simulink model "ddc_bpm_476_066_hw_cosim"  (Simulink 7.8)
settings: Solver=ode45  StartTime=0.0  StopTime=200e-4  RelTol=1e-3
undefined symbols (not defined in the file): A, dt_sim, frev_476, Fs_adc, N
libraries: simulink x3, xbsIndex_r4 x1, JTAGRuntimeCosim_r4 x1
settings Model: Creator=lucas.russo  LastModifiedBy=lucas.russo

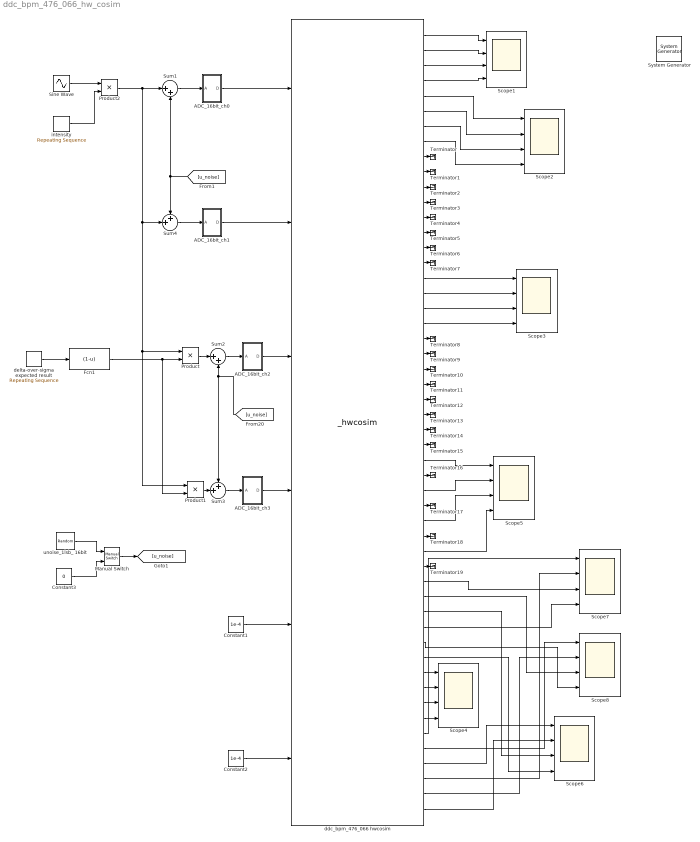
== system ddc_bpm_476_066_hw_cosim ==
  " System Generator" : xbsIndex_r4/ System Generator  Tag=genX  xilinxfamily=virtex6  part=xc6vlx240t  speed=-1  package=ff1156  synthesis_tool=XST  clock_wrapper=Clock Enables  directory=./netlistJTAG_COsim_ddc_bpm_476_066  proj_type=Project Navigator  Synth_file=XST Defaults  Impl_file=ISE Defaults  testbench=on  simulink_period=dt_sim  sysclk_period=10  dcm_input_clock_period=10  incr_netlist=off  trim_vbits=Everywhere in SubSystem  dbl_ovrd=According to Block Masks  core_generation=According to Block Masks  run_coregen=off  deprecated_control=off  eval_field=0  block_type=sysgen
  ADC_16bit_ch0 : Subsystem
  ADC_16bit_ch1 : Subsystem
  ADC_16bit_ch2 : Subsystem
  ADC_16bit_ch3 : Subsystem
  Constant1 : Constant  Value=1e-4  OutDataTypeStr=fixdt(1,26,22)
  Constant2 : Constant  Value=1e-4  OutDataTypeStr=fixdt(1,26,22)
  Constant3 : Constant  Value=0  SampleTime=0
  Fcn1 : Fcn  Expr=(1-u)
  Manual Switch : simulink/Signal Routing/Manual Switch  sw=1  action=0  varsize=off
  Product : Product  RndMeth=Zero
  Product1 : Product  RndMeth=Zero
  Product2 : Product  RndMeth=Zero
  Scope{1..8} (8 alike) : Scope  NumInputPorts=4
      Scope1 settings: TimeRange=4.726537192257835e-007  YMin=4.34876e-005~0.463882~0.00990226~4.5e-005  YMax=4.80652e-005~0.512712~0.0111025~9.5e-005  MaxDataPoints=1000000
      Scope2 settings: TimeRange=4.726537192257835e-007  YMin=4.34876e-005~0.463882~0.00990226~4.5e-005  YMax=4.80652e-005~0.512712~0.0111025~9.5e-005  MaxDataPoints=1000000
      Scope3 settings: TimeRange=4.726537192257835e-007  YMin=4.34876e-005~0.463882~0.00990226~4.5e-005  YMax=4.80652e-005~0.512712~0.0111025~9.5e-005  SaveName=ScopeData2  MaxDataPoints=1000000
      Scope4 settings: TimeRange=4.726537192257835e-007  YMin=4.34876e-005~0.463882~0.00990226~4.5e-005  YMax=4.80652e-005~0.512712~0.0111025~9.5e-005  SaveName=ScopeData3  MaxDataPoints=1000000
      Scope5 settings: TimeRange=4.726537192257835e-007  YMin=4.34876e-005~0.463882~0.00990226~4.5e-005  YMax=4.80652e-005~0.512712~0.0111025~9.5e-005  SaveName=ScopeData4  MaxDataPoints=1000000
      Scope6 settings: TimeRange=4.726537192257835e-007  YMin=4.34876e-005~0.463882~0.00990226~4.5e-005  YMax=4.80652e-005~0.512712~0.0111025~9.5e-005  SaveName=ScopeData5  MaxDataPoints=1000000
      Scope7 settings: TimeRange=4.726537192257835e-007  YMin=4.34876e-005~1.14441e-005~0.00990226~4.5e-005  YMax=4.80652e-005~1.14441e-005~0.0111025~9.5e-005  SaveName=ScopeData6  MaxDataPoints=1000000
      Scope8 settings: TimeRange=4.726537192257835e-007  YMin=4.34876e-005~-3.75509e-007~0.00990226~4.5e-005  YMax=4.80652e-005~-3.39747e-007~0.0111025~9.5e-005  SaveName=ScopeData7  MaxDataPoints=1000000
  Sine Wave : Sin  Frequency=2*pi*frev_476  SampleTime=0
  Sum1 : Sum  Inputs=|++
  Sum2 : Sum  Inputs=|++
  Sum3 : Sum  Inputs=++|
  Sum4 : Sum  Inputs=++|
  Terminator{,1..19} (20 alike) : Terminator
  ddc_bpm_476_066 hwcosim : JTAGRuntimeCosim_r4/_hwcosim  clkSrc=Single Stepped  hasCombinationalPath=on  bitfileName=D:\Sysgen_projects\ddc_bpm_476_066\models\netlistJTAG_COsim_ddc_bpm_476_066_v2_3\ddc_bpm_476_066_cw.bit  skipConfig=off  cable=Auto Detect  speed=N/A  cablePort=N/A  cableLocation=Local  shareCable=off  enable_codebug=on  design_xtable=|  engineDll=JTAGCosimEngine.dll  cableWaitTime=10  bscanPos=-1  IRLengths=[]  useWaitBox=1  hasBufgmux=on  Scheme=Cosim  useCmdProc=1  hasProc=0  block_type=jtagcosim
      | {
      |   'clkWrapper' => 'ddc_bpm_476_066_cw',
      |   'clocksGcd' => 1,
      |   'device' => 'xc6vlx240t-1ff1156',
      |   'ports' => {
      |     'adc_ch0_dbg_data_o' => {
      |       'bd_port_index' => 0,
      |       'direction' => 'out',
      |       'icon_text' => 'adc_ch0_dbg_data_o',
      |       'period' => 1,
      |       'proxy_name' => 'ddc_bpm_476_066/BPF/adc_ch0_dbg_data_o',
      |       'sim_pause_trigger' => false,
      |       'type' => 'Fix_16_15',
      |       'width' => 16,
      |     },
      |     'adc_ch0_i' => {
      |       'bd_port_index' => 0,
      |       'direction' => 'in',
      |       'icon_text' => 'adc_ch0_i',
      |       'period' => 1,
      |       'proxy_name' => 'ddc_bpm_476_066/adc_ch0_i',
      |       'sim_pause_trigger' => false,
      |       'type' => 'Fix_16_15',
      |       'width' => 16,
      |     },
      |     'adc_ch1_dbg_data_o' => {
      |       'bd_port_index' => 1,
      |       'direction' => 'out',
      |       'icon_text' => 'adc_ch1_dbg_data_o',
      |       'period' => 1,
      |       'proxy_name' => 'ddc_bpm_476_066/BPF/adc_ch1_dbg_data_o',
      |       'sim_pause_trigger' => false,
      |       'type' => 'Fix_16_15',
      |       'width' => 16,
      |     },
      |     'adc_ch1_i' => {
      |       'bd_port_index' => 1,
      |       'direction' => 'in',
      |       'icon_text' => 'adc_ch1_i',
      |       'period' => 1,
      |       'proxy_name' => 'ddc_bpm_476_066/adc_ch1_i',
      |       'sim_pause_trigger' => false,
      |       'type' => 'Fix_16_15',
      |       'width' => 16,
      |     },
      |     'adc_ch2_dbg_data_o' => {
      |       'bd_port_index' => 2,
      |       'direction' => 'out',
      |       'icon_text' => 'adc_ch2_dbg_data_o',
      |       'period' => 1,
      |       'proxy_name' => 'ddc_bpm_476_066/BPF/adc_ch2_dbg_data_o',
      |       'sim_pause_trigger' => false,
      |       'type' => 'Fix_16_15',
      |       'width' => 16,
      |     },
      |     'adc_ch2_i' => {
      |       'bd_port_index' => 2,
      |       'direction' => 'in',
      |       'icon_text' => 'adc_ch2_i',
      |       'period' => 1,
      |       'proxy_name' => 'ddc_bpm_476_066/adc_ch2_i',
      |       'sim_pause_trigger' => false,
      |       'type' => 'Fix_16_15',
      |       'width' => 16,
      |     },
      |     'adc_ch3_dbg_data_o' => {
      |       'bd_port_index' => 3,
      |       'direction' => 'out',
      |       'icon_text' => 'adc_ch3_dbg_data_o',
      |       'period' => 1,
      |       'proxy_name' => 'ddc_bpm_476_066/BPF/adc_ch3_dbg_data_o',
      |       'sim_pause_trigger' => false,
      |       'type' => 'Fix_16_15',
      |       'width' => 16,
      |     },
      |     'adc_ch3_i' => {
      |       'bd_port_index' => 3,
      |       'direction' => 'in',
      |       'icon_text' => 'adc_ch3_i',
      |       'period' => 1,
      |       'proxy_name' => 'ddc_bpm_476_066/adc_ch3_i',
      |       'sim_pause_trigger' => false,
      |       'type' => 'Fix_16_15',
      |       'width' => 16,
      |     },
      |     'bpf_ch0_o' => {
      |       'bd_port_index' => 4,
      |       'direction' => 'out',
      |       'icon_text' => 'bpf_ch0_o',
      |       'period' => 1,
      |       'proxy_name' => 'ddc_bpm_476_066/BPF/bpf_ch0_o',
      |       'sim_pause_trigger' => false,
      |       'type' => 'Fix_24_22',
      |       'width' => 24,
      |     },
      |     'bpf_ch1_o' => {
      |       'bd_port_index' => 5,
      |       'direction' => 'out',
      |       'icon_text' => 'bpf_ch1_o',
      |       'period' => 1,
      |       'proxy_name' => 'ddc_bpm_476_066/BPF/bpf_ch1_o',
      |       'sim_pause_trigger' => false,
      |       'type' => 'Fix_24_22',
      |       'width' => 24,
      |     },
      |     'bpf_ch2_o' => {
      |       'bd_port_index' => 6,
      |       'direction' => 'out',
      |       'icon_text' => 'bpf_ch2_o',
      |       'period' => 1,
      |       'proxy_name' => 'ddc_bpm_476_066/BPF/bpf_ch2_o',
      |       'sim_pause_trigger' => false,
      |       'type' => 'Fix_24_22',
      |       'width' => 24,
      |     },
      |     'bpf_ch3_o' => {
      |       'bd_port_index' => 7,
      |       'direction' => 'out',
      |       'icon_text' => 'bpf_ch3_o',
      |       'period' => 1,
      |       'proxy_name' => 'ddc_bpm_476_066/BPF/bpf_ch3_o',
      |       'sim_pause_trigger' => false,
      |       'type' => 'Fix_24_22',
      |       'width' => 24,
      |     },
      |     'cic_fofb_ch0_i_o' => {
      |       'bd_port_index' => 8,
      |       'direction' => 'out',
      |       'icon_text' => 'cic_fofb_ch0_i_o',
      |       'period' => 1113,
      |       'proxy_name' => 'ddc_bpm_476_066/Channel0_fofb/cic_fofb_ch0_i_o',
      |       'sim_pause_trigger' => false,
      |       'type' => 'Fix_25_23',
      |       'width' => 25,
      |     },
      |     'cic_fofb_ch0_q_o' => {
      |       'bd_port_index' => 9,
      |       'direction' => 'out',
      |       'icon_text' => 'cic_fofb_ch0_q_o',
      |       'period' => 1113,
      |       'proxy_name' => 'ddc_bpm_476_066/Channel0_fofb/cic_fofb_ch0_q_o',
      |       'sim_pause_trigger' => false,
      |       'type' => 'Fix_25_23',
      |       'width' => 25,
      |     },
      |     'cic_fofb_ch1_i_o' => {
      |       'bd_port_index' => 10,
      |       'direction' => 'out',
      |       'icon_text' => 'cic_fofb_ch1_i_o',
      |       'period' => 1113,
      |       'proxy_name' => 'ddc_bpm_476_066/Channel1_fofb/cic_fofb_ch1_i_o',
      |       'sim_pause_trigger' => false,
      |       'type' => 'Fix_25_23',
      |       'width' => 25,
      |     },
      |     'cic_fofb_ch1_q_o' => {
      |       'bd_port_index' => 11,
      |       'direction' => 'out',
      |       'icon_text' => 'cic_fofb_ch1_q_o',
      |       'period' => 1113,
      |       'proxy_name' => 'ddc_bpm_476_066/Channel1_fofb/cic_fofb_ch1_q_o',
      |       'sim_pause_trigger' => false,
      |       'type' => 'Fix_25_23',
      |       'width' => 25,
      |     },
      |     'cic_fofb_ch2_i_o' => {
      |       'bd_port_index' => 12,
      |       'direction' => 'out',
      |       'icon_text' => 'cic_fofb_ch2_i_o',
      |       'period' => 1113,
      |       'proxy_name' => 'ddc_bpm_476_066/Channel2_fofb/cic_fofb_ch2_i_o',
      |       'sim_pause_trigger' => false,
      |       'type' => 'Fix_25_23',
      |       'width' => 25,
      |     },
      |     'cic_fofb_ch2_q_o' => {
      |       'bd_port_index' => 13,
      |       'direction' => 'out',
      |       'icon_text' => 'cic_fofb_ch2_q_o',
      |       'period' => 1113,
      |       'proxy_name' => 'ddc_bpm_476_066/Channel2_fofb/cic_fofb_ch2_q_o',
      |       'sim_pause_trigger' => false,
      |       'type' => 'Fix_25_23',
      |       'width' => 25,
      |     },
      |     'cic_fofb_ch3_i_o' => {
      |       'bd_port_index' => 14,
      |       'direction' => 'out',
      |       'icon_text' => 'cic_fofb_ch3_i_o',
      |       'period' => 1113,
      |       'proxy_name' => 'ddc_bpm_476_066/Channel3_fofb/cic_fofb_ch3_i_o',
      |       'sim_pause_trigger' => false,
      |       'type' => 'Fix_25_23',
      |       'width' => 25,
      |     },
      |     'cic_fofb_ch3_q_o' => {
      |       'bd_port_index' => 15,
      |       'direction' => 'out',
      |       'icon_text' => 'cic_fofb_ch3_q_o',
      |       'period' => 1113,
      |       'proxy_name' => 'ddc_bpm_476_066/Channel3_fofb/cic_fofb_ch3_q_o',
      |       'sim_pause_trigger' => false,
      |       'type' => 'Fix_25_23',
      |       'width' => 25,
      |     },
      |     'del_sig_div_fofb_thres_i' => {
      |       'bd_port_index' => 4,
      |       'direction' => 'in',
      |       'icon_text' => 'del_sig_div_fofb_thres_i',
      |       'period' => 1,
      |       'proxy_name' => 'ddc_bpm_476_066/del_sig_div_fofb_thres_i',
      |       'sim_pause_trigger' => false,
      |       'type' => 'Fix_27_23',
      |       'width' => 27,
      |     },
      |     'del_sig_div_tbt_thres_i' => {
      |       'bd_port_index' => 5,
      |       'direction' => 'in',
      |       'icon_text' => 'del_sig_div_tbt_thres_i',
      |       'period' => 1,
      |       'proxy_name' => 'ddc_bpm_476_066/del_sig_div_tbt_thres_i',
      |       'sim_pause_trigger' => false,
      |       'type' => 'Fix_27_23',
      |       'width' => 27,
      |     },
      |     'fofb_amp_ch0_o' => {
      |       'bd_port_index' => 16,
      |       'direction' => 'out',
      |       'icon_text' => 'fofb_amp_ch0_o',
      |       'period' => 1113,
      |       'proxy_name' => 'ddc_bpm_476_066/Channel0_fofb/fofb_amp_ch0_o',
      |       'sim_pause_trigger' => false,
      |       'type' => 'Fix_25_23',
      |       'width' => 25,
      |     },
      |     'fofb_amp_ch1_o' => {
      |       'bd_port_index' => 17,
      |       'direction' => 'out',
      |       'icon_text' => 'fofb_amp_ch1_o',
      |       'period' => 1113,
      |       'proxy_name' => 'ddc_bpm_476_066/Channel1_fofb/fofb_amp_ch1_o',
      |       'sim_pause_trigger' => false,
      |       'type' => 'Fix_25_23',
      |       'width' => 25,
      |     },
      |     'fofb_amp_ch2_o' => {
      |       'bd_port_index' => 18,
      |       'direction' => 'out',
      |       'icon_text' => 'fofb_amp_ch2_o',
      |       'period' => 1113,
      |       'proxy_name' => 'ddc_bpm_476_066/Channel2_fofb/fofb_amp_ch2_o',
      |       'sim_pause_trigger' => false,
      |       'type' => 'Fix_25_23',
      |       'width' => 25,
      |     },
      |     'fofb_amp_ch3_o' => {
      |       'bd_port_index' => 19,
      |       'direction' => 'out',
      |       'icon_text' => 'fofb_amp_ch3_o',
      |       'period' => 1113,
      |       'proxy_name' => 'ddc_bpm_476_066/Channel3_fofb/fofb_amp_ch3_o',
      |       'sim_pause_trigger' => false,
      |       'type' => 'Fix_25_23',
      |       'width' => 25,
      |     },
      |     'mix_ch0_i_o' => {
      |       'bd_port_index' => 20,
      |       'direction' => 'out',
      |       'icon_text' => 'mix_ch0_i_o',
      |       'period' => 1,
      |       'proxy_name' => 'ddc_bpm_476_066/Channel0_tbt/mix_ch0_i_o',
      |       'sim_pause_trigger' => false,
      |       'type' => 'Fix_24_22',
      |       'width' => 24,
      |     },
      |     'mix_ch0_q_o' => {
      |       'bd_port_index' => 21,
      |       'direction' => 'out',
      |       'icon_text' => 'mix_ch0_q_o',
      |       'period' => 1,
      |       'proxy_name' => 'ddc_bpm_476_066/Channel0_tbt/mix_ch0_q_o',
      |       'sim_pause_trigger' => false,
      |       'type' => 'Fix_24_22',
      |       'width' => 24,
      |     },
      |     'mix_ch1_i_o' => {
      |       'bd_port_index' => 22,
      |       'direction' => 'out',
      |       'icon_text' => 'mix_ch1_i_o',
      |       'period' => 1,
      |       'proxy_name' => 'ddc_bpm_476_066/Channel1_tbt/mix_ch1_i_o',
      |       'sim_pause_trigger' => false,
      |       'type' => 'Fix_24_22',
      |       'width' => 24,
      |     },
      |     'mix_ch1_q_o' => {
      |       'bd_port_index' => 23,
      |       'direction' => 'out',
      |       'icon_text' => 'mix_ch1_q_o',
      |       'period' => 1,
      |       'proxy_name' => 'ddc_bpm_476_066/Channel1_tbt/mix_ch1_q_o',
      |       'sim_pause_trigger' => false,
      |       'type' => 'Fix_24_22',
      |       'width' => 24,
      |     },
      |     'mix_ch2_i_o' => {
      |       'bd_port_index' => 24,
      |       'direction' => 'out',
      |       'icon_text' => 'mix_ch2_i_o',
      |       'period' => 1,
      |       'proxy_name' => 'ddc_bpm_476_066/Channel2_tbt/mix_ch2_i_o',
      |       'sim_pause_trigger' => false,
      |       'type' => 'Fix_24_22',
      |       'width' => 24,
      |     },
      |     'mix_ch2_q_o' => {
      |       'bd_port_index' => 25,
      |       'direction' => 'out',
      |       'icon_text' => 'mix_ch2_q_o',
      |       'period' => 1,
      |       'proxy_name' => 'ddc_bpm_476_066/Channel2_tbt/mix_ch2_q_o',
      |       'sim_pause_trigger' => false,
      |       'type' => 'Fix_24_22',
      |       'width' => 24,
      |     },
      |     'mix_ch3_i_o' => {
      |       'bd_port_index' => 26,
      |       'direction' => 'out',
      |       'icon_text' => 'mix_ch3_i_o',
      |       'period' => 1,
      |       'proxy_name' => 'ddc_bpm_476_066/Channel3_tbt/mix_ch3_i_o',
      |       'sim_pause_trigger' => false,
      |       'type' => 'Fix_24_22',
      |       'width' => 24,
      |     },
      |     'mix_ch3_q_o' => {
      |       'bd_port_index' => 27,
      |       'direction' => 'out',
      |       'icon_text' => 'mix_ch3_q_o',
      |       'period' => 1,
      |       'proxy_name' => 'ddc_bpm_476_066/Channel3_tbt/mix_ch3_q_o',
      |       'sim_pause_trigger' => false,
      |       'type' => 'Fix_24_22',
      |       'width' => 24,
      |     },
      |     'poly35_ch0_i_o' => {
      |       'bd_port_index' => 28,
      |       'direction' => 'out',
      |       'icon_text' => 'poly35_ch0_i_o',
      |       'period' => 35,
      |       'proxy_name' => 'ddc_bpm_476_066/Channel0_tbt/poly35_ch0_i_o',
      |       'sim_pause_trigger' => false,
      |       'type' => 'Fix_25_23',
      |       'width' => 25,
      |     },
      |     'poly35_ch0_q_o' => {
      |       'bd_port_index' => 29,
      |       'direction' => 'out',
      |       'icon_text' => 'poly35_ch0_q_o',
      |       'period' => 35,
      |       'proxy_name' => 'ddc_bpm_476_066/Channel0_tbt/poly35_ch0_q_o',
      |       'sim_pause_trigger' => false,
      |       'type' => 'Fix_25_23',
      |       'width' => 25,
      |     },
      |     'poly35_ch1_i_o' => {
      |       'bd_port_index' => 30,
      |       'direction' => 'out',
      |       'icon_text' => 'poly35_ch1_i_o',
      |       'period' => 35,
      |       'proxy_name' => 'ddc_bpm_476_066/Channel1_tbt/poly35_ch1_i_o',
      |       'sim_pause_trigger' => false,
      |       'type' => 'Fix_25_23',
      |       'width' => 25,
      |     },
      |     'poly35_ch1_q_o' => {
      |       'bd_port_index' => 31,
      |       'direction' => 'out',
      |       'icon_text' => 'poly35_ch1_q_o',
      |       'period' => 35,
      |       'proxy_name' => 'ddc_bpm_476_066/Channel1_tbt/poly35_ch1_q_o',
      |       'sim_pause_trigger' => false,
      |       'type' => 'Fix_25_23',
      |       'width' => 25,
      |     },
      |     'poly35_ch2_i_o' => {
      |       'bd_port_index' => 32,
      |       'direction' => 'out',
      |       'icon_text' => 'poly35_ch2_i_o',
      |       'period' => 35,
      |       'proxy_name' => 'ddc_bpm_476_066/Channel2_tbt/poly35_ch2_i_o',
      |       'sim_pause_trigger' => false,
      |       'type' => 'Fix_25_23',
      |       'width' => 25,
      |     },
      |     'poly35_ch2_q_o' => {
      |       'bd_port_index' => 33,
      |       'direction' => 'out',
      |       'icon_text' => 'poly35_ch2_q_o',
      |       'period' => 35,
      |       'proxy_name' => 'ddc_bpm_476_066/Channel2_tbt/poly35_ch2_q_o',
      |       'sim_pause_trigger' => false,
      |       'type' => 'Fix_25_23',
      |       'width' => 25,
      |     },
      |     'poly35_ch3_i_o' => {
      |       'bd_port_index' => 34,
      |       'direction' => 'out',
      |       'icon_text' => 'poly35_ch3_i_o',
      |       'period' => 35,
      |       'proxy_name' => 'ddc_bpm_476_066/Channel3_tbt/poly35_ch3_i_o',
      |       'sim_pause_trigger' => false,
      |       'type' => 'Fix_25_23',
      |       'width' => 25,
      |     },
      |     'poly35_ch3_q_o' => {
      |       'bd_port_index' => 35,
      |       'direction' => 'out',
      |       'icon_text' => 'poly35_ch3_q_o',
      |       'period' => 35,
      |       'proxy_name' => 'ddc_bpm_476_066/Channel3_tbt/poly35_ch3_q_o',
      |       'sim_pause_trigger' => false,
      |       'type' => 'Fix_25_23',
      |       'width' => 25,
      |     },
      |     'q_fofb_o' => {
      |       'bd_port_index' => 36,
      |       'direction' => 'out',
      |       'icon_text' => 'q_fofb_o',
      |       'period' => 1,
      |       'proxy_name' => 'ddc_bpm_476_066/q_fofb_o',
      |       'sim_pause_trigger' => false,
      |       'type' => 'Fix_24_23',
      |       'width' => 24,
      |     },
      |     'q_monit_o' => {
      |       'bd_port_index' => 37,
      |       'direction' => 'out',
      |       'icon_text' => 'q_monit_o',
      |       'period' => 11130000,
      |       'proxy_name' => 'ddc_bpm_476_066/q_monit_o',
      |       'sim_pause_trigger' => false,
      |       'type' => 'Fix_24_23',
      |       'width' => 24,
      |     },
      |     'q_tbt_o' => {
      |       'bd_port_index' => 38,
      |       'direction' => 'out',
      |       'icon_text' => 'q_tbt_o',
      |       'period' => 1,
      |       'proxy_name' => 'ddc_bpm_476_066/q_tbt_o',
      |       'sim_pause_trigger' => false,
      |       'type' => 'Fix_24_23',
      |       'width' => 24,
      |     },
      |     'sum_fofb_o' => {
      |       'bd_port_index' => 39,
      |       'direction' => 'out',
      |       'icon_text' => 'sum_fofb_o',
      |       'period' => 1,
      |       'proxy_name' => 'ddc_bpm_476_066/sum_fofb_o',
      |       'sim_pause_trigger' => false,
      |       'type' => 'Fix_24_20',
      |       'width' => 24,
      |     },
      |     'sum_monit_o' => {
      |       'bd_port_index' => 40,
      |       'direction' => 'out',
      |       'icon_text' => 'sum_monit_o',
      |       'period' => 11130000,
      |       'proxy_name' => 'ddc_bpm_476_066/sum_monit_o',
      |       'sim_pause_trigger' => false,
      |       'type' => 'Fix_24_20',
      |       'width' => 24,
      |     },
      |     'sum_tbt_o' => {
      |       'bd_port_index' => 41,
      |       'direction' => 'out',
      |       'icon_text' => 'sum_tbt_o',
      |       'period' => 1,
      |       'proxy_name' => 'ddc_bpm_476_066/sum_tbt_o',
      |       'sim_pause_trigger' => false,
      |       'type' => 'Fix_24_20',
      |       'width' => 24,
      |     },
      |     'tbt_amp_ch0_o' => {
      |       'bd_port_index' => 42,
      |       'direction' => 'out',
      |       'icon_text' => 'tbt_amp_ch0_o',
      |       'period' => 35,
      |       'proxy_name' => 'ddc_bpm_476_066/Channel0_tbt/tbt_amp_ch0_o',
      |       'sim_pause_trigger' => false,
      |       'type' => 'Fix_25_23',
      |       'width' => 25,
      |     },
      |     'tbt_amp_ch1_o' => {
      |       'bd_port_index' => 43,
      |       'direction' => 'out',
      |       'icon_text' => 'tbt_amp_ch1_o',
      |       'period' => 35,
      |       'proxy_name' => 'ddc_bpm_476_066/Channel1_tbt/tbt_amp_ch1_o',
      |       'sim_pause_trigger' => false,
      |       'type' => 'Fix_25_23',
      |       'width' => 25,
      |     },
      |     'tbt_amp_ch2_o' => {
      |       'bd_port_index' => 44,
      |       'direction' => 'out',
      |       'icon_text' => 'tbt_amp_ch2_o',
      |       'period' => 35,
      |       'proxy_name' => 'ddc_bpm_476_066/Channel2_tbt/tbt_amp_ch2_o',
      |       'sim_pause_trigger' => false,
      |       'type' => 'Fix_25_23',
      |       'width' => 25,
      |     },
      |     'tbt_amp_ch3_o' => {
      |       'bd_port_index' => 45,
      |       'direction' => 'out',
      |       'icon_text' => 'tbt_amp_ch3_o',
      |       'period' => 35,
      |       'proxy_name' => 'ddc_bpm_476_066/Channel3_tbt/tbt_amp_ch3_o',
      |       'sim_pause_trigger' => false,
      |       'type' => 'Fix_25_23',
      |       'width' => 25,
      |     },
      |     'x_fofb_o' => {
      |       'bd_port_index' => 46,
      |       'direction' => 'out',
      |       'icon_text' => 'x_fofb_o',
      |       'period' => 1,
      |       'proxy_name' => 'ddc_bpm_476_066/x_fofb_o',
      |       'sim_pause_trigger' => false,
      |       'type' => 'Fix_24_23',
      |       'width' => 24,
      |     },
      |     'x_monit_o' => {
      |       'bd_port_index' => 47,
      |       'direction' => 'out',
      |       'icon_text' => 'x_monit_o',
      |       'period' => 11130000,
      |       'proxy_name' => 'ddc_bpm_476_066/x_monit_o',
      |       'sim_pause_trigger' => false,
      |       'type' => 'Fix_24_23',
      |       'width' => 24,
      |     },
      |     'x_tbt_o' => {
      |       'bd_port_index' => 48,
      |       'direction' => 'out',
      |       'icon_text' => 'x_tbt_o',
      |       'period' => 1,
      |       'proxy_name' => 'ddc_bpm_476_066/x_tbt_o',
      |       'sim_pause_trigger' => false,
      |       'type' => 'Fix_24_23',
      |       'width' => 24,
      |     },
      |     'y_fofb_o' => {
      |       'bd_port_index' => 49,
      |       'direction' => 'out',
      |       'icon_text' => 'y_fofb_o',
      |       'period' => 1,
      |       'proxy_name' => 'ddc_bpm_476_066/y_fofb_o',
      |       'sim_pause_trigger' => false,
      |       'type' => 'Fix_24_23',
      |       'width' => 24,
      |     },
      |     'y_monit_o' => {
      |       'bd_port_index' => 50,
      |       'direction' => 'out',
      |       'icon_text' => 'y_monit_o',
      |       'period' => 11130000,
      |       'proxy_name' => 'ddc_bpm_476_066/y_monit_o',
      |       'sim_pause_trigger' => false,
      |       'type' => 'Fix_24_23',
      |       'width' => 24,
      |     },
      |     'y_tbt_o' => {
      |       'bd_port_index' => 51,
      |       'direction' => 'out',
      |       'icon_text' => 'y_tbt_o',
      |       'period' => 1,
      |       'proxy_name' => 'ddc_bpm_476_066/y_tbt_o',
      |       'sim_pause_trigger' => false,
      |       'type' => 'Fix_24_23',
      |       'width' => 24,
      |     },
      |   },
      |   'shared_memories' => {},
      | }
  delta-over-sigma expected result : simulink/Sources/Repeating Sequence  rep_seq_t=[0 10e-4 10e-4 20e-4 20e-4 30e-4 30e-4 40e-4]  rep_seq_y=vrms_att
  intensity : simulink/Sources/Repeating Sequence  rep_seq_t=[0 1e-4 1e-4 2e-4 2e-4 3e-4 3e-4 4e-4]  rep_seq_y=[1 1 1 1 1 1 1 1]
  unoise_1lsb_ 16bit : UniformRandomNumber  Minimum=-0.5*(2/2^16)  Maximum=0.5*(2/2^16)  Seed=4517861  SampleTime=0
  wires:
  Sine Wave/1 -> Product2/1
  Product2/1 -> Sum1/1, Product/1, Product1/1, Sum4/2
  intensity/1 -> Product2/2
  ADC_16bit_ch0/1(D) -> ddc_bpm_476_066 hwcosim/1
  ADC_16bit_ch1/1(D) -> ddc_bpm_476_066 hwcosim/2
  ADC_16bit_ch2/1(D) -> ddc_bpm_476_066 hwcosim/3
  ADC_16bit_ch3/1(D) -> ddc_bpm_476_066 hwcosim/4
  Constant1/1 -> ddc_bpm_476_066 hwcosim/5
  Constant2/1 -> ddc_bpm_476_066 hwcosim/6
  delta-over-sigma expected result/1 -> Fcn1/1
  Fcn1/1 -> Product/2, Product1/2
  unoise_1lsb_ 16bit/1 -> Manual Switch/1
  Constant3/1 -> Manual Switch/2
  Manual Switch/1 -> [u_noise]
  [u_noise] -> Sum2/2, Sum3/1
  Product/1 -> Sum2/1
  Sum2/1 -> ADC_16bit_ch2/1(A)
  Product1/1 -> Sum3/2
  Sum3/1 -> ADC_16bit_ch3/1(A)
  [u_noise] -> Sum1/2, Sum4/1
  Sum1/1 -> ADC_16bit_ch0/1(A)
  Sum4/1 -> ADC_16bit_ch1/1(A)
  ddc_bpm_476_066 hwcosim/1 -> Scope1/1
  ddc_bpm_476_066 hwcosim/2 -> Scope1/2
  ddc_bpm_476_066 hwcosim/3 -> Scope1/3
  ddc_bpm_476_066 hwcosim/4 -> Scope1/4
  ddc_bpm_476_066 hwcosim/5 -> Scope2/1
  ddc_bpm_476_066 hwcosim/6 -> Scope2/2
  ddc_bpm_476_066 hwcosim/7 -> Scope2/3
  ddc_bpm_476_066 hwcosim/8 -> Scope2/4
  ddc_bpm_476_066 hwcosim/17 -> Scope3/1
  ddc_bpm_476_066 hwcosim/18 -> Scope3/2
  ddc_bpm_476_066 hwcosim/19 -> Scope3/3
  ddc_bpm_476_066 hwcosim/20 -> Scope3/4
  ddc_bpm_476_066 hwcosim/29 -> Scope5/1
  ddc_bpm_476_066 hwcosim/31 -> Scope5/2
  ddc_bpm_476_066 hwcosim/33 -> Scope5/3
  ddc_bpm_476_066 hwcosim/35 -> Scope5/4
  ddc_bpm_476_066 hwcosim/49 -> Scope6/1
  ddc_bpm_476_066 hwcosim/52 -> Scope6/2
  ddc_bpm_476_066 hwcosim/39 -> Scope6/3
  ddc_bpm_476_066 hwcosim/42 -> Scope6/4
  ddc_bpm_476_066 hwcosim/43 -> Scope4/1
  ddc_bpm_476_066 hwcosim/44 -> Scope4/2
  ddc_bpm_476_066 hwcosim/45 -> Scope4/3
  ddc_bpm_476_066 hwcosim/46 -> Scope4/4
  ddc_bpm_476_066 hwcosim/37 -> Scope7/3
  ddc_bpm_476_066 hwcosim/50 -> Scope7/2
  ddc_bpm_476_066 hwcosim/47 -> Scope7/1
  ddc_bpm_476_066 hwcosim/40 -> Scope7/4
  ddc_bpm_476_066 hwcosim/38 -> Scope8/3
  ddc_bpm_476_066 hwcosim/48 -> Scope8/1
  ddc_bpm_476_066 hwcosim/51 -> Scope8/2
  ddc_bpm_476_066 hwcosim/41 -> Scope8/4
  ddc_bpm_476_066 hwcosim/9 -> Terminator/1
  ddc_bpm_476_066 hwcosim/10 -> Terminator1/1
  ddc_bpm_476_066 hwcosim/11 -> Terminator2/1
  ddc_bpm_476_066 hwcosim/12 -> Terminator3/1
  ddc_bpm_476_066 hwcosim/13 -> Terminator4/1
  ddc_bpm_476_066 hwcosim/14 -> Terminator5/1
  ddc_bpm_476_066 hwcosim/15 -> Terminator6/1
  ddc_bpm_476_066 hwcosim/16 -> Terminator7/1
  ddc_bpm_476_066 hwcosim/21 -> Terminator8/1
  ddc_bpm_476_066 hwcosim/22 -> Terminator9/1
  ddc_bpm_476_066 hwcosim/23 -> Terminator10/1
  ddc_bpm_476_066 hwcosim/24 -> Terminator11/1
  ddc_bpm_476_066 hwcosim/25 -> Terminator12/1
  ddc_bpm_476_066 hwcosim/26 -> Terminator13/1
  ddc_bpm_476_066 hwcosim/27 -> Terminator14/1
  ddc_bpm_476_066 hwcosim/28 -> Terminator15/1
  ddc_bpm_476_066 hwcosim/30 -> Terminator16/1
  ddc_bpm_476_066 hwcosim/32 -> Terminator17/1
  ddc_bpm_476_066 hwcosim/34 -> Terminator18/1
  ddc_bpm_476_066 hwcosim/36 -> Terminator19/1

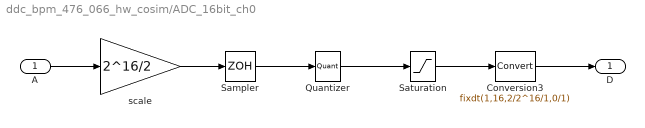
== system ddc_bpm_476_066_hw_cosim/ADC_16bit_ch0 ==
  A : Inport  OutDataTypeStr=double
  Conversion3 : DataTypeConversion  OutDataTypeStr=fixdt(1,16,2/2^16/1,0/1)  ConvertRealWorld=Stored Integer (SI)  LockScale=on
  Quantizer : Quantizer  QuantizationInterval=1  SampleTime=dt_sim
  Sampler : ZeroOrderHold  SampleTime=1/Fs_adc
  Saturation : Saturate  UpperLimit=65536/2-1  LowerLimit=-65536/2  OutDataTypeStr=Inherit: Inherit via back propagation
  scale : Gain  Gain=2^16/2  SaturateOnIntegerOverflow=on  OutDataTypeStr=Inherit: Same as input  ParamDataTypeStr=Inherit: Same as input
  D : Outport
  wires:
  A/1 -> scale/1
  Conversion3/1 -> D/1
  Quantizer/1 -> Saturation/1
  Sampler/1 -> Quantizer/1
  Saturation/1 -> Conversion3/1
  scale/1 -> Sampler/1

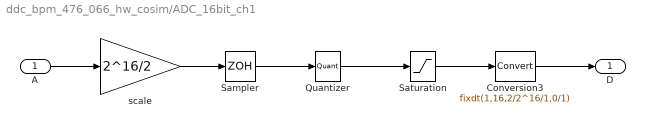
== system ddc_bpm_476_066_hw_cosim/ADC_16bit_ch1 ==
  A : Inport  OutDataTypeStr=double
  Conversion3 : DataTypeConversion  OutDataTypeStr=fixdt(1,16,2/2^16/1,0/1)  ConvertRealWorld=Stored Integer (SI)  LockScale=on
  Quantizer : Quantizer  QuantizationInterval=1  SampleTime=dt_sim
  Sampler : ZeroOrderHold  SampleTime=1/Fs_adc
  Saturation : Saturate  UpperLimit=65536/2-1  LowerLimit=-65536/2  OutDataTypeStr=Inherit: Inherit via back propagation
  scale : Gain  Gain=2^16/2  SaturateOnIntegerOverflow=on  OutDataTypeStr=Inherit: Same as input  ParamDataTypeStr=Inherit: Same as input
  D : Outport
  wires:
  A/1 -> scale/1
  Conversion3/1 -> D/1
  Quantizer/1 -> Saturation/1
  Sampler/1 -> Quantizer/1
  Saturation/1 -> Conversion3/1
  scale/1 -> Sampler/1

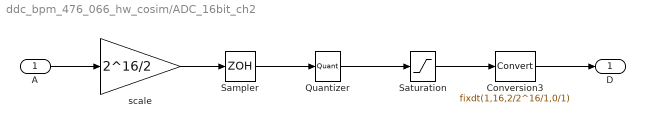
== system ddc_bpm_476_066_hw_cosim/ADC_16bit_ch2 ==
  A : Inport  OutDataTypeStr=double
  Conversion3 : DataTypeConversion  OutDataTypeStr=fixdt(1,16,2/2^16/1,0/1)  ConvertRealWorld=Stored Integer (SI)  LockScale=on
  Quantizer : Quantizer  QuantizationInterval=1  SampleTime=dt_sim
  Sampler : ZeroOrderHold  SampleTime=1/Fs_adc
  Saturation : Saturate  UpperLimit=65536/2-1  LowerLimit=-65536/2  OutDataTypeStr=Inherit: Inherit via back propagation
  scale : Gain  Gain=2^16/2  SaturateOnIntegerOverflow=on  OutDataTypeStr=Inherit: Same as input  ParamDataTypeStr=Inherit: Same as input
  D : Outport
  wires:
  A/1 -> scale/1
  Conversion3/1 -> D/1
  Quantizer/1 -> Saturation/1
  Sampler/1 -> Quantizer/1
  Saturation/1 -> Conversion3/1
  scale/1 -> Sampler/1

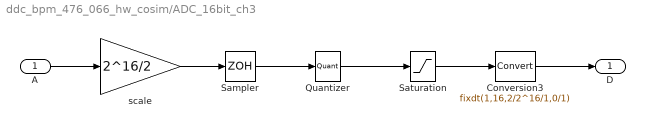
== system ddc_bpm_476_066_hw_cosim/ADC_16bit_ch3 ==
  A : Inport  OutDataTypeStr=double
  Conversion3 : DataTypeConversion  OutDataTypeStr=fixdt(1,16,2/2^16/1,0/1)  ConvertRealWorld=Stored Integer (SI)  LockScale=on
  Quantizer : Quantizer  QuantizationInterval=1  SampleTime=dt_sim
  Sampler : ZeroOrderHold  SampleTime=1/Fs_adc
  Saturation : Saturate  UpperLimit=65536/2-1  LowerLimit=-65536/2  OutDataTypeStr=Inherit: Inherit via back propagation
  scale : Gain  Gain=2^16/2  SaturateOnIntegerOverflow=on  OutDataTypeStr=Inherit: Same as input  ParamDataTypeStr=Inherit: Same as input
  D : Outport
  wires:
  A/1 -> scale/1
  Conversion3/1 -> D/1
  Quantizer/1 -> Saturation/1
  Sampler/1 -> Quantizer/1
  Saturation/1 -> Conversion3/1
  scale/1 -> Sampler/1
